simulink model "ControleFF_trajetoria_D"  (R2020a)
settings: Solver=ode23  StartTime=0.0  StopTime=60  FixedStep=rate  RelTol=1e-3
values from neighbouring files (symbols this model uses):
  Beff = 50    [controle.m]    (also in controle_FF.m; controle_PD.m)
  Jeff = 2.2    [controle.m]    (also in controle_FF.m = 0.5; controle_PD.m = 0.5)
  K = 17.7    [controle.m]    (also in controle_FF.m = 0.785398163397; controle_PD.m = 0.785398163397)
  Kd = (2*zeta*wn*Jeff - Beff)/K    (= -2.32768361582)    [controle.m]    (also in controle_FF.m = -44.5633840657; controle_PD.m = -44.5633840657)
  Kp = (wn^2*Jeff)/K    (= 0.497175141243)    [controle.m]    (also in controle_FF.m = 143.239448783; controle_PD.m = 143.239448783)
  N = 10    [controle.m]    (also in controle_FF.m = 3; controle_PD.m = 3)
  r = 1/100    (= 0.01)    [controle.m]    (also in controle_FF.m = 1./[231.22*4 139.138 139.138 231.22 231.22]; controle_PD.m = 1./[231.22*4 139.138 139.138 231.22 231.22])
  SP_theta = [0;0;0;0;0]    [controle.m]    (also in controle_FF.m = [0 0 0 0 0]; controle_PD.m)
libraries: simulink_extras x6
(part 1 of 5)
settings Model: Creator=Karoline  LastModifiedBy=lunet
settings DataIOCC: ReturnWorkspaceOutputs=off
settings DebuggingCC: ArithmeticOperatorsInVariantConditions=warning
settings SFSimCC: SimUseLocalCustomCode=off  CustomCodeUndefinedFunction=UseInterfaceOnly
settings RTWCC: RTWUseLocalCustomCode=off
settings CodeAppCC: StateflowObjectComments=on

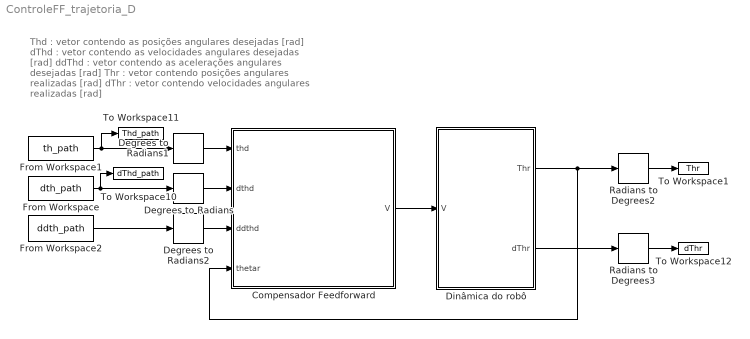
== system ControleFF_trajetoria_D ==
  note: Thd : vetor contendo as posições angulares desejadas [rad]
      | dThd : vetor contendo as velocidades angulares desejadas [rad]
      | ddThd : vetor contendo as acelerações angulares desejadas [rad]
      |
      | Thr : vetor contendo posições angulares realizadas [rad]
      | dThr : vetor contendo velocidades angulares realizadas [rad]
  Compensador Feedforward : Subsystem
  Degrees to Radians : simulink_extras/Transformations/Degrees to Radians
  Degrees to Radians1 : simulink_extras/Transformations/Degrees to Radians
  Degrees to Radians2 : simulink_extras/Transformations/Degrees to Radians
  Dinâmica do robô : Subsystem
  From Workspace : FromWorkspace  VariableName=dth_path
  From Workspace1 : FromWorkspace  VariableName=th_path
  From Workspace2 : FromWorkspace  VariableName=ddth_path
  Radians to Degrees2 : simulink_extras/Transformations/Radians to Degrees
  Radians to Degrees3 : simulink_extras/Transformations/Radians to Degrees
  To Workspace1 : ToWorkspace  VariableName=Thr  SaveFormat=Structure With Time  SampleTime=-1
  To Workspace10 : ToWorkspace  VariableName=dThd_path  SaveFormat=Structure With Time  SampleTime=-1
  To Workspace11 : ToWorkspace  VariableName=Thd_path  SaveFormat=Structure With Time  SampleTime=-1
  To Workspace12 : ToWorkspace  VariableName=dThr  SaveFormat=Structure With Time  SampleTime=-1
  wires:
  Dinâmica do robô/2("dThr ") -> Radians to Degrees3/1
  Compensador Feedforward/1(V) -> Dinâmica do robô/1(V)
  Dinâmica do robô/1(Thr) -> Compensador Feedforward/4(thetar), Radians to Degrees2/1
  From Workspace2/1 -> Degrees to Radians2/1
  Degrees to Radians2/1 -> Compensador Feedforward/3(ddthd)
  From Workspace/1 -> Degrees to Radians/1, To Workspace10/1
  From Workspace1/1 -> Degrees to Radians1/1, To Workspace11/1
  Degrees to Radians1/1 -> Compensador Feedforward/1(thd)
  Degrees to Radians/1 -> Compensador Feedforward/2(dthd)
  Radians to Degrees3/1 -> To Workspace12/1
  Radians to Degrees2/1 -> To Workspace1/1

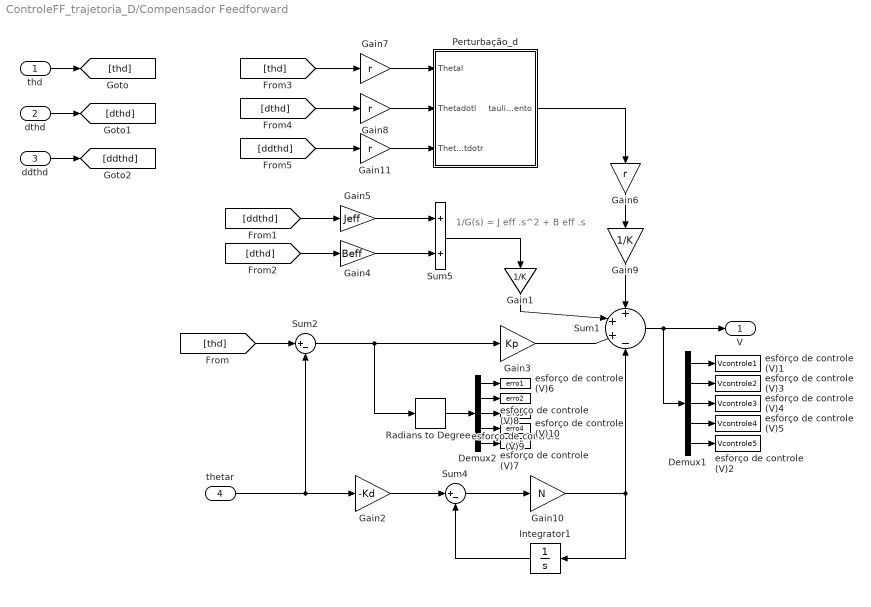
== system ControleFF_trajetoria_D/Compensador Feedforward ==
  note: 1/G(s) = J eff .s^2 + B eff .s
  thd : Inport
  dthd : Inport  Port=2
  ddthd : Inport  Port=3
  thetar : Inport  Port=4
  Demux1 : Demux  Outputs=5
  Demux2 : Demux  Outputs=5
  Gain1 : Gain  Gain=1/K
  Gain10 : Gain  Gain=N
  Gain{6..8,11} (4 alike) : Gain  Gain=r
  Gain2 : Gain  Gain=-Kd
  Gain3 : Gain  Gain=Kp
  Gain4 : Gain  Gain=Beff
  Gain5 : Gain  Gain=Jeff
  Gain9 : Gain  Gain=1/K
  Integrator1 : Integrator
  Perturbação_d : Subsystem
  Radians to Degrees : simulink_extras/Transformations/Radians to Degrees
  Sum1 : Sum  Inputs=+|+|+|-
  Sum2 : Sum  Inputs=|+-
  Sum4 : Sum  Inputs=|+-
  Sum5 : Sum
  esforço de controle (V)1 : ToWorkspace  VariableName=Vcontrole1  SampleTime=-1
  esforço de controle (V)10 : ToWorkspace  VariableName=erro4  SampleTime=-1
  esforço de controle (V)2 : ToWorkspace  VariableName=Vcontrole5  SampleTime=-1
  esforço de controle (V)3 : ToWorkspace  VariableName=Vcontrole2  SampleTime=-1
  esforço de controle (V)4 : ToWorkspace  VariableName=Vcontrole3  SampleTime=-1
  esforço de controle (V)5 : ToWorkspace  VariableName=Vcontrole4  SampleTime=-1
  esforço de controle (V)6 : ToWorkspace  VariableName=erro1  SampleTime=-1
  esforço de controle (V)7 : ToWorkspace  VariableName=erro5  SampleTime=-1
  esforço de controle (V)8 : ToWorkspace  VariableName=erro2  SampleTime=-1
  esforço de controle (V)9 : ToWorkspace  VariableName=erro3  SampleTime=-1
  V : Outport  VectorParamsAs1DForOutWhenUnconnected=off
  wires:
  Gain2/1 -> Sum4/1
  thetar/1 -> Sum2/2, Gain2/1
  Sum4/1 -> Gain10/1
  Integrator1/1 -> Sum4/2
  Gain10/1 -> Sum1/4, Integrator1/1
  Gain4/1 -> Sum5/2
  Gain5/1 -> Sum5/1
  Sum5/1 -> Gain1/1
  Gain8/1 -> Perturbação_d/2(Thetadotl)
  Gain7/1 -> Perturbação_d/1(Thetal)
  [thd] -> Gain7/1
  [dthd] -> Gain8/1
  Perturbação_d/1(tauligamento) -> Gain6/1
  Gain6/1 -> Gain9/1
  Gain9/1 -> Sum1/1
  thd/1 -> [thd]
  [thd] -> Sum2/1
  ddthd/1 -> [ddthd]
  [ddthd] -> Gain5/1
  dthd/1 -> [dthd]
  [dthd] -> Gain4/1
  Gain3/1 -> Sum1/3
  Gain1/1 -> Sum1/2
  Demux1/1 -> esforço de controle (V)1/1
  Demux1/5 -> esforço de controle (V)2/1
  Demux1/4 -> esforço de controle (V)5/1
  Sum1/1 -> Demux1/1, V/1
  Demux1/2 -> esforço de controle (V)3/1
  Demux1/3 -> esforço de controle (V)4/1
  Demux2/5 -> esforço de controle (V)7/1
  Demux2/4 -> esforço de controle (V)10/1
  Demux2/1 -> esforço de controle (V)6/1
  Sum2/1 -> Radians to Degrees/1, Gain3/1
  Demux2/2 -> esforço de controle (V)8/1
  Demux2/3 -> esforço de controle (V)9/1
  Radians to Degrees/1 -> Demux2/1
  [ddthd] -> Gain11/1
  Gain11/1 -> Perturbação_d/3(Thetadotdotr)

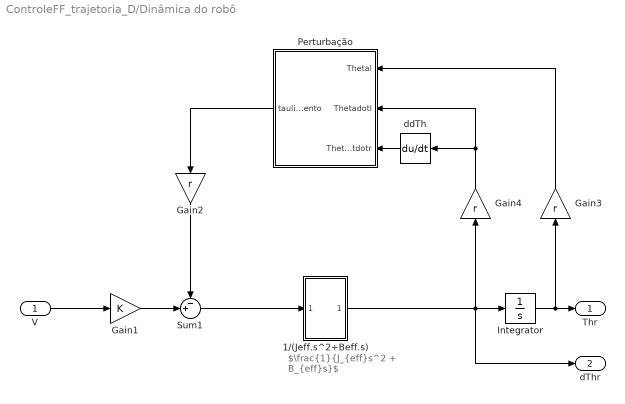
== system ControleFF_trajetoria_D/Dinâmica do robô ==
  note: $\frac{1}{J_{eff}s^2 + B_{eff}s}$
  V : Inport
  1/(Jeff.s^2+Beff.s) : Subsystem
  Gain1 : Gain  Gain=K
  Gain2 : Gain  Gain=r
  Gain3 : Gain  Gain=r
  Gain4 : Gain  Gain=r
  Integrator : Integrator  InitialCondition=SP_theta*pi/180
  Perturbação : Subsystem
  Sum1 : Sum  Inputs=-+|
  ddTh : Derivative
  Thr : Outport  VectorParamsAs1DForOutWhenUnconnected=off
  "dThr " : Outport  Port=2  VectorParamsAs1DForOutWhenUnconnected=off
  wires:
  Perturbação/1(tauligamento) -> Gain2/1
  Gain1/1 -> Sum1/2
  Integrator/1 -> Thr/1, Gain3/1
  V/1 -> Gain1/1
  Gain2/1 -> Sum1/1
  ddTh/1 -> Perturbação/3(Thetadotdotr)
  Gain3/1 -> Perturbação/1(Thetal)
  Gain4/1 -> ddTh/1, Perturbação/2(Thetadotl)
  1/(Jeff.s^2+Beff.s)/1(Out1) -> Integrator/1, "dThr "/1, Gain4/1
  Sum1/1 -> 1/(Jeff.s^2+Beff.s)/1(In1)

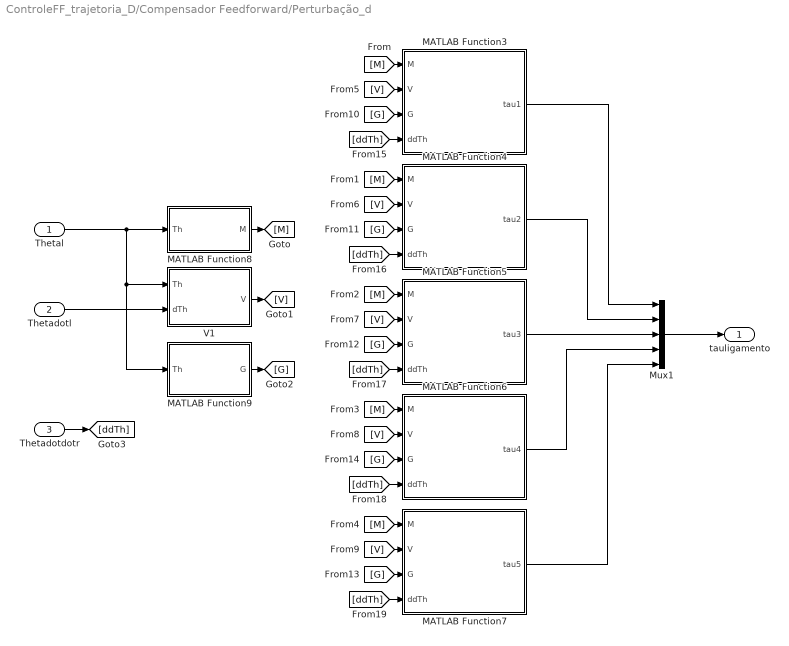
== system ControleFF_trajetoria_D/Compensador Feedforward/Perturbação_d ==
  Thetal : Inport
  Thetadotl : Inport  Port=2
  Thetadotdotr : Inport  Port=3
  MATLAB Function3 : MATLAB Function  TreatAsAtomicUnit=on
  MATLAB Function4 : MATLAB Function  TreatAsAtomicUnit=on
  MATLAB Function5 : MATLAB Function  TreatAsAtomicUnit=on
  MATLAB Function6 : MATLAB Function  TreatAsAtomicUnit=on
  MATLAB Function7 : MATLAB Function  TreatAsAtomicUnit=on
  MATLAB Function8 : MATLAB Function  TreatAsAtomicUnit=on
  MATLAB Function9 : MATLAB Function  TreatAsAtomicUnit=on
  Mux1 : Mux  Inputs=5
  V1 : MATLAB Function  TreatAsAtomicUnit=on
  tauligamento : Outport  VectorParamsAs1DForOutWhenUnconnected=off
  wires:
  [G] -> MATLAB Function6/3(G)
  MATLAB Function8/1(M) -> [M]
  [M] -> MATLAB Function6/1(M)
  [M] -> MATLAB Function4/1(M)
  [M] -> MATLAB Function3/1(M)
  Thetal/1 -> MATLAB Function8/1(Th), MATLAB Function9/1(Th), V1/1(Th)
  [ddTh] -> MATLAB Function5/4(ddTh)
  [V] -> MATLAB Function3/2(V)
  [ddTh] -> MATLAB Function3/4(ddTh)
  [G] -> MATLAB Function7/3(G)
  [ddTh] -> MATLAB Function6/4(ddTh)
  [V] -> MATLAB Function6/2(V)
  Thetadotl/1 -> V1/2(dTh)
  [G] -> MATLAB Function5/3(G)
  [G] -> MATLAB Function3/3(G)
  [G] -> MATLAB Function4/3(G)
  MATLAB Function9/1(G) -> [G]
  [V] -> MATLAB Function7/2(V)
  [ddTh] -> MATLAB Function4/4(ddTh)
  [V] -> MATLAB Function5/2(V)
  [V] -> MATLAB Function4/2(V)
  V1/1(V) -> [V]
  [M] -> MATLAB Function7/1(M)
  [M] -> MATLAB Function5/1(M)
  [ddTh] -> MATLAB Function7/4(ddTh)
  Mux1/1 -> tauligamento/1
  MATLAB Function3/1(tau1) -> Mux1/1
  MATLAB Function4/1(tau2) -> Mux1/2
  MATLAB Function5/1(tau3) -> Mux1/3
  MATLAB Function6/1(tau4) -> Mux1/4
  MATLAB Function7/1(tau5) -> Mux1/5
  Thetadotdotr/1 -> [ddTh]

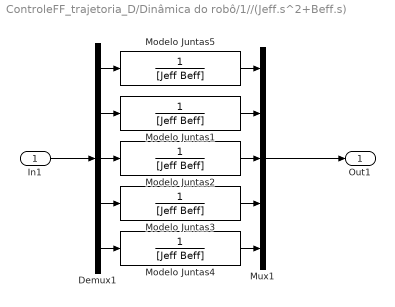
== system ControleFF_trajetoria_D/Dinâmica do robô/1//(Jeff.s^2+Beff.s) ==
  In1 : Inport
  Demux1 : Demux  Outputs=5
  Modelo Juntas{1..5} (5 alike) : TransferFcn  Denominator=[Jeff Beff]
  Mux1 : Mux  Inputs=5
  Out1 : Outport
  wires:
  Modelo Juntas5/1 -> Mux1/1
  Modelo Juntas3/1 -> Mux1/4
  Demux1/1 -> Modelo Juntas5/1
  Modelo Juntas2/1 -> Mux1/3
  Demux1/3 -> Modelo Juntas2/1
  Modelo Juntas1/1 -> Mux1/2
  Demux1/5 -> Modelo Juntas4/1
  Demux1/2 -> Modelo Juntas1/1
  Demux1/4 -> Modelo Juntas3/1
  Modelo Juntas4/1 -> Mux1/5
  Mux1/1 -> Out1/1
  In1/1 -> Demux1/1

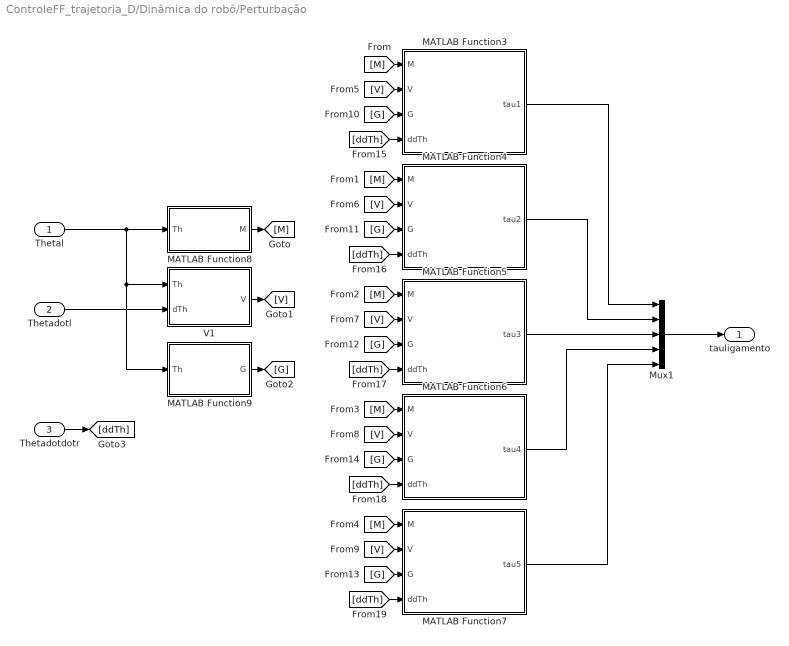
== system ControleFF_trajetoria_D/Dinâmica do robô/Perturbação ==
  Thetal : Inport
  Thetadotl : Inport  Port=2
  Thetadotdotr : Inport  Port=3
  MATLAB Function3 : MATLAB Function  TreatAsAtomicUnit=on
  MATLAB Function4 : MATLAB Function  TreatAsAtomicUnit=on
  MATLAB Function5 : MATLAB Function  TreatAsAtomicUnit=on
  MATLAB Function6 : MATLAB Function  TreatAsAtomicUnit=on
  MATLAB Function7 : MATLAB Function  TreatAsAtomicUnit=on
  MATLAB Function8 : MATLAB Function  TreatAsAtomicUnit=on
  MATLAB Function9 : MATLAB Function  TreatAsAtomicUnit=on
  Mux1 : Mux  Inputs=5
  V1 : MATLAB Function  TreatAsAtomicUnit=on
  tauligamento : Outport  VectorParamsAs1DForOutWhenUnconnected=off
  wires:
  [G] -> MATLAB Function6/3(G)
  MATLAB Function8/1(M) -> [M]
  [M] -> MATLAB Function6/1(M)
  [M] -> MATLAB Function4/1(M)
  [M] -> MATLAB Function3/1(M)
  Thetal/1 -> MATLAB Function8/1(Th), MATLAB Function9/1(Th), V1/1(Th)
  [ddTh] -> MATLAB Function5/4(ddTh)
  [V] -> MATLAB Function3/2(V)
  [ddTh] -> MATLAB Function3/4(ddTh)
  [G] -> MATLAB Function7/3(G)
  [ddTh] -> MATLAB Function6/4(ddTh)
  [V] -> MATLAB Function6/2(V)
  Thetadotl/1 -> V1/2(dTh)
  [G] -> MATLAB Function5/3(G)
  [G] -> MATLAB Function3/3(G)
  [G] -> MATLAB Function4/3(G)
  MATLAB Function9/1(G) -> [G]
  [V] -> MATLAB Function7/2(V)
  [ddTh] -> MATLAB Function4/4(ddTh)
  [V] -> MATLAB Function5/2(V)
  [V] -> MATLAB Function4/2(V)
  V1/1(V) -> [V]
  [M] -> MATLAB Function7/1(M)
  [M] -> MATLAB Function5/1(M)
  [ddTh] -> MATLAB Function7/4(ddTh)
  Mux1/1 -> tauligamento/1
  MATLAB Function3/1(tau1) -> Mux1/1
  MATLAB Function4/1(tau2) -> Mux1/2
  MATLAB Function5/1(tau3) -> Mux1/3
  MATLAB Function6/1(tau4) -> Mux1/4
  MATLAB Function7/1(tau5) -> Mux1/5
  Thetadotdotr/1 -> [ddTh]

== matlab function ControleFF_trajetoria_D/Compensador Feedforward/Perturbação_d/MATLAB Function4 ==
  data: M input; V input; tau2 output; G input; ddTh input
function tau2  = calcul_dk2(M, V, G, ddTh)

tau2 = M(2,1)*ddTh(1) + M(2,3)*ddTh(3) + M(2,4)*ddTh(4) + M(2,5)*ddTh(5) ...
       + V(2) + G(2);

== matlab function ControleFF_trajetoria_D/Compensador Feedforward/Perturbação_d/MATLAB Function5 ==
  data: M input; V input; tau3 output; G input; ddTh input
function tau3  = calcul_dk3(M, V, G, ddTh)

tau3 = M(3,1)*ddTh(1) + M(3,2)*ddTh(2) + M(3,4)*ddTh(4) + M(3,5)*ddTh(5) ...
       + V(3) + G(3);

== matlab function ControleFF_trajetoria_D/Compensador Feedforward/Perturbação_d/MATLAB Function6 ==
  data: M input; V input; tau4 output; G input; ddTh input
function tau4 = calcul_dk4(M, V, G, ddTh)

tau4 = M(4,1)*ddTh(1) + M(4,2)*ddTh(2) + M(4,3)*ddTh(3) + M(4,5)*ddTh(5) ...
       + V(4) + G(4);

== matlab function ControleFF_trajetoria_D/Compensador Feedforward/Perturbação_d/MATLAB Function7 ==
  data: M input; V input; tau5 output; G input; ddTh input
function tau5  = calcul_dk5(M, V, G, ddTh)

tau5 = M(5,1)*ddTh(1) + M(5,2)*ddTh(2) + M(5,3)*ddTh(3) + M(5,4)*ddTh(4) ...
       + V(5) + G(5);

== matlab function ControleFF_trajetoria_D/Compensador Feedforward/Perturbação_d/MATLAB Function8 ==
  data: Th input; M output
function M = calcul_M(Th)

th1 = Th(1);
th2 = Th(2);
th3 = Th(3);
th4 = Th(4);
th5 = Th(5);

M = [ (87*cos(th2)^2*cos(th5))/2500 + (87*cos(th3)^2*cos(th5))/2500 - (33*cos(th2)^2*sin(th3))/50 + (53231*cos(th2)^2)/62500 + (8453*cos(th3)^2)/31250 - (9*cos(th5)^2)/3200 - (8453*cos(th2)^2*cos(th3)^2)/15625 - (217*cos(th2)^2*cos(th4)^2)/80000 + (9*cos(th2)^2*cos(th5)^2)/3200 - (217*cos(th3)^2*cos(th4)^2)/80000 + (9*cos(th3)^2*cos(th5)^2)/3200 - (87*cos(th2)^2*cos(th3)^2*cos(th5))/1250 - (33*cos(th2)*cos(th3)*sin(th2))/50 + (217*cos(th2)^2*cos(th3)^2*cos(th4)^2)/40000 - (9*cos(th2)^2*cos(th3)^2*cos(th5)^2)/1600 + (9*cos(th2)^2*cos(th4)^2*cos(th5)^2)/3200 + (9*cos(th3)^2*cos(th4)^2*cos(th5)^2)/3200 - (3*cos(th2)^2*cos(th5)*sin(th3))/80 - (9*cos(th2)^2*cos(th3)^2*cos(th4)^2*cos(th5)^2)/1600 - (3*cos(th2)*cos(th3)*cos(th5)*sin(th2))/80 + (8453*cos(th2)*cos(th3)*sin(th2)*sin(th3))/15625 - (87*cos(th2)*cos(th4)*sin(th2)*sin(th5))/2500 - (87*cos(th3)*cos(th4)*sin(th3)*sin(th5))/2500 - (3*cos(th2)^2*cos(th3)*cos(th4)*sin(th5))/80 + (3*cos(th2)*cos(th4)*sin(th2)*sin(th3)*sin(th5))/80 - (217*cos(th2)*cos(th3)*cos(th4)^2*sin(th2)*sin(th3))/40000 + (9*cos(th2)*cos(th3)*cos(th5)^2*sin(th2)*sin(th3))/1600 + (87*cos(th2)*cos(th3)^2*cos(th4)*sin(th2)*sin(th5))/1250 + (87*cos(th2)^2*cos(th3)*cos(th4)*sin(th3)*sin(th5))/1250 + (87*cos(th2)*cos(th3)*cos(th5)*sin(th2)*sin(th3))/1250 - (9*cos(th2)*cos(th4)*cos(th5)*sin(th2)*sin(th5))/1600 - (9*cos(th3)*cos(th4)*cos(th5)*sin(th3)*sin(th5))/1600 + (9*cos(th2)*cos(th3)*cos(th4)^2*cos(th5)^2*sin(th2)*sin(th3))/1600 + (9*cos(th2)*cos(th3)^2*cos(th4)*cos(th5)*sin(th2)*sin(th5))/800 + (9*cos(th2)^2*cos(th3)*cos(th4)*cos(th5)*sin(th3)*sin(th5))/800 + 3793/80000, -(sin(th4)*(1500*sin(th2)*sin(th5) - 217*cos(th2)*cos(th4)*sin(th3) - 217*cos(th3)*cos(th4)*sin(th2) + 1392*cos(th2)*cos(th3)*sin(th5) - 1392*sin(th2)*sin(th3)*sin(th5) + 225*cos(th2)*cos(th3)*cos(th5)*sin(th5) - 225*cos(th5)*sin(th2)*sin(th3)*sin(th5) + 225*cos(th2)*cos(th4)*cos(th5)^2*sin(th3) + 225*cos(th3)*cos(th4)*cos(th5)^2*sin(th2)))/80000, (sin(th4)*(217*cos(th2)*cos(th4)*sin(th3) + 217*cos(th3)*cos(th4)*sin(th2) - 1392*cos(th2)*cos(th3)*sin(th5) + 1392*sin(th2)*sin(th3)*sin(th5) - 225*cos(th2)*cos(th3)*cos(th5)*sin(th5) + 225*cos(th5)*sin(th2)*sin(th3)*sin(th5) - 225*cos(th2)*cos(th4)*cos(th5)^2*sin(th3) - 225*cos(th3)*cos(th4)*cos(th5)^2*sin(th2)))/80000, (489*cos(th2)*cos(th3))/80000 - (489*sin(th2)*sin(th3))/80000 - (3*cos(th2)*cos(th4)*sin(th5))/160 - (9*cos(th2)*cos(th3)*cos(th5)^2)/3200 + (9*cos(th5)^2*sin(th2)*sin(th3))/3200 + (87*cos(th2)*cos(th4)*sin(th3)*sin(th5))/5000 + (87*cos(th3)*cos(th4)*sin(th2)*sin(th5))/5000 + (9*cos(th2)*cos(th4)*cos(th5)*sin(th3)*sin(th5))/3200 + (9*cos(th3)*cos(th4)*cos(th5)*sin(th2)*sin(th5))/3200, (sin(th4)*(353*cos(th2)*sin(th3) + 353*cos(th3)*sin(th2) - 1500*cos(th2)*cos(th5) + 1392*cos(th2)*cos(th5)*sin(th3) + 1392*cos(th3)*cos(th5)*sin(th2)))/80000;
                                                                                                                                                                                                                                                                                                                                                                                                                                                                                                                                                                                                                                                                                                                                                                                                                                                                                                                                                                                                                                                                                                                                                                                                                                                                                                                                                                                                                                                                                                                                                                                            -(sin(th4)*(1500*sin(th2)*sin(th5) - 217*cos(th2)*cos(th4)*sin(th3) - 217*cos(th3)*cos(th4)*sin(th2) + 1392*cos(th2)*cos(th3)*sin(th5) - 1392*sin(th2)*sin(th3)*sin(th5) + 225*cos(th2)*cos(th3)*cos(th5)*sin(th5) - 225*cos(th5)*sin(th2)*sin(th3)*sin(th5) + 225*cos(th2)*cos(th4)*cos(th5)^2*sin(th3) + 225*cos(th3)*cos(th4)*cos(th5)^2*sin(th2)))/80000,                                                                                                                                                                                                                       (87*cos(th5))/2500 - (33*sin(th3))/50 - (3*cos(th5)*sin(th3))/80 + (217*cos(th4)^2)/80000 + (9*cos(th5)^2)/3200 - (9*cos(th4)^2*cos(th5)^2)/3200 - (3*cos(th3)*cos(th4)*sin(th5))/80 + 54781/62500,                                                                                                                                                                                   (87*cos(th5))/2500 - (33*sin(th3))/100 - (3*cos(th5)*sin(th3))/160 + (217*cos(th4)^2)/80000 + (9*cos(th5)^2)/3200 - (9*cos(th4)^2*cos(th5)^2)/3200 - (3*cos(th3)*cos(th4)*sin(th5))/160 + 72749/250000,                                                                                                                                                                                                                                                                                                                                                                                                                     -(3*sin(th4)*sin(th5)*(75*cos(th5) - 500*sin(th3) + 464))/80000,                                                          (353*cos(th4))/80000 - (3*cos(th3)*sin(th5))/160 + (87*cos(th4)*cos(th5))/5000 - (3*cos(th4)*cos(th5)*sin(th3))/160;
                                                                                                                                                                                                                                                                                                                                                                                                                                                                                                                                                                                                                                                                                                                                                                                                                                                                                                                                                                                                                                                                                                                                                                                                                                                                                                                                                                                                                                                                                                                                                                                                                            (sin(th4)*(217*cos(th2)*cos(th4)*sin(th3) + 217*cos(th3)*cos(th4)*sin(th2) - 1392*cos(th2)*cos(th3)*sin(th5) + 1392*sin(th2)*sin(th3)*sin(th5) - 225*cos(th2)*cos(th3)*cos(th5)*sin(th5) + 225*cos(th5)*sin(th2)*sin(th3)*sin(th5) - 225*cos(th2)*cos(th4)*cos(th5)^2*sin(th3) - 225*cos(th3)*cos(th4)*cos(th5)^2*sin(th2)))/80000,                                                                                                                                                                                                                   (87*cos(th5))/2500 - (33*sin(th3))/100 - (3*cos(th5)*sin(th3))/160 + (217*cos(th4)^2)/80000 + (9*cos(th5)^2)/3200 - (9*cos(th4)^2*cos(th5)^2)/3200 - (3*cos(th3)*cos(th4)*sin(th5))/160 + 72749/250000,                                                                                                                                                                                                                                                                                          (87*cos(th5))/2500 + (217*cos(th4)^2)/80000 + (9*cos(th5)^2)/3200 - (9*cos(th4)^2*cos(th5)^2)/3200 + 72749/250000,                                                                                                                                                                                                                                                                                                                                                                                                                                       -(3*sin(th4)*sin(th5)*(75*cos(th5) + 464))/80000,                                                                                                                                                         (cos(th4)*(1392*cos(th5) + 353))/80000;
                                                                                                                                                                                                                                                                                                                                                                                                                                                                                                                                                                                                                                                                                                                                                                                                                                                                                                                                                                                                                                                                                                                                                                                                                                                                                                                                                                                                                                                                                                                                                      (489*cos(th2)*cos(th3))/80000 - (489*sin(th2)*sin(th3))/80000 - (3*cos(th2)*cos(th4)*sin(th5))/160 - (9*cos(th2)*cos(th3)*cos(th5)^2)/3200 + (9*cos(th5)^2*sin(th2)*sin(th3))/3200 + (87*cos(th2)*cos(th4)*sin(th3)*sin(th5))/5000 + (87*cos(th3)*cos(th4)*sin(th2)*sin(th5))/5000 + (9*cos(th2)*cos(th4)*cos(th5)*sin(th3)*sin(th5))/3200 + (9*cos(th3)*cos(th4)*cos(th5)*sin(th2)*sin(th5))/3200,                                                                                                                                                                                                                                                                                                                                                                               -(3*sin(th4)*sin(th5)*(75*cos(th5) - 500*sin(th3) + 464))/80000,                                                                                                                                                                                                                                                                                                                                                                 -(3*sin(th4)*sin(th5)*(75*cos(th5) + 464))/80000,                                                                                                                                                                                                                                                                                                                                                                                                                                                              489/80000 - (9*cos(th5)^2)/3200,                                                                                                                                                                                                    0;
                                                                                                                                                                                                                                                                                                                                                                                                                                                                                                                                                                                                                                                                                                                                                                                                                                                                                                                                                                                                                                                                                                                                                                                                                                                                                                                                                                                                                                                                                                                                                                                                                                                                                                                                                                                                                                                 (sin(th4)*(353*cos(th2)*sin(th3) + 353*cos(th3)*sin(th2) - 1500*cos(th2)*cos(th5) + 1392*cos(th2)*cos(th5)*sin(th3) + 1392*cos(th3)*cos(th5)*sin(th2)))/80000,                                                                                                                                                                                                                                                                                                               (353*cos(th4))/80000 - (3*cos(th3)*sin(th5))/160 + (87*cos(th4)*cos(th5))/5000 - (3*cos(th4)*cos(th5)*sin(th3))/160,                                                                                                                                                                                                                                                                                                                                                                              (cos(th4)*(1392*cos(th5) + 353))/80000,                                                                                                                                                                                                                                                                                                                                                                                                                                                                                               0,                                                                                                                                                                                            353/80000];

== matlab function ControleFF_trajetoria_D/Compensador Feedforward/Perturbação_d/MATLAB Function9 ==
  data: Th input; G output
function G = calcul_G(Th)

g = 9.80665;
th1 = Th(1);
th2 = Th(2);
th3 = Th(3);
th4 = Th(4);
th5 = Th(5);

G = [                                                                                                                                                                                                                                                                                               0;
 -g*((49*cos(th2)*sin(th3))/125 - cos(th2)/2 + (49*cos(th3)*sin(th2))/125 + (3*cos(th2)*cos(th5)*sin(th3))/40 + (3*cos(th3)*cos(th5)*sin(th2))/40 + (3*cos(th2)*cos(th3)*cos(th4)*sin(th5))/40 - (3*cos(th4)*sin(th2)*sin(th3)*sin(th5))/40);
                 -g*((49*cos(th2)*sin(th3))/125 + (49*cos(th3)*sin(th2))/125 + (3*cos(th2)*cos(th5)*sin(th3))/40 + (3*cos(th3)*cos(th5)*sin(th2))/40 + (3*cos(th2)*cos(th3)*cos(th4)*sin(th5))/40 - (3*cos(th4)*sin(th2)*sin(th3)*sin(th5))/40);
                                                                                                                                                                                                                                                (3*g*sin(th4)*sin(th5)*sin(th2 + th3))/40;
                                                                                       -g*((3*cos(th2)*cos(th3)*sin(th5))/40 - (3*sin(th2)*sin(th3)*sin(th5))/40 + (3*cos(th2)*cos(th4)*cos(th5)*sin(th3))/40 + (3*cos(th3)*cos(th4)*cos(th5)*sin(th2))/40)];
